simulink library "tqd"  (R2021b)
settings: Solver=VariableStepAuto  StartTime=0.0  StopTime=10.0  RelTol=1e-3
undefined symbols (not defined in the file or in its folder): ATQD_BOSEnBPSPosn_X_kph, ATQD_BOSMap_X_rpm, ATQD_BOSMap_Y_pct, ATQD_CreepBaseTqD_X_kph, ATQD_CreepBaseTqD_Y_Deg, ATQD_CreepBaseTqR_X_kph, ATQD_CreepBaseTqR_Y_Deg, ATQD_CreepBPSDisPosn_X_Deg, ATQD_CreepBPSDisPosnR_X_Deg, ATQD_CreepBPSEnPosn_X_Deg, ATQD_CreepBPSEnPosnR_X_Deg, ATQD_CreepDeltaTq_X_kph, ATQD_CreepIterm_X_kph, ATQD_CreepIterm_Y_kph, ATQD_CreepItermMaxLimit_X_pct, ATQD_CreepPreloadTime_X_kph, ATQD_CreepPreloadTq_X_kph, ATQD_CreepPreloadTq_Y_s, ATQD_CreepProtTq_X_Deg, ATQD_CreepPterm_X_kph, ATQD_ECOTqMapD_X_rpm, ATQD_ECOTqMapD_Y_pct, ATQD_NL1TqMapD_X_rpm, ATQD_NL1TqMapD_Y_pct, ATQD_NRMRrEDUSpRat_X_rpm, ATQD_NRMRrEDUSpRat_Y_Nm, ATQD_PedalMapClimbUpLim_X_rpm, ATQD_PedalMapClimbUpLim_Y_Deg, ATQD_PreLoadTq_X_s, ATQD_SL1TqMapD_X_rpm, ATQD_SL1TqMapD_Y_pct, ATQD_WhlTqCapMotGain_X_pct, ATQD_WhlTqCapMotGain_Y_mV, ENUM_ACCPEDALLOWSW_LOWIDLE, ENUM_ACCPEDALLOWSW_NOIDLE, ENUM_CHRGPLUGSTA_NONE, ENUM_CRASHSTATE_NOCRASH, ENUM_DCDCFAULTSTA_WORKING, ENUM_DRIVEMODE_ECO, ENUM_DRIVEMODE_NRM, ENUM_DRIVEMODE_SPORT, ENUM_DRIVETRAIN_AWD, ENUM_DRIVETRAIN_FWD, ENUM_DRIVETRAIN_RWD, ENUM_EBSBRKSW_PRESSED, ENUM_EBSTORQUERWQ_LIMIT, ENUM_EBSTORQUERWQ_TORQUE, ENUM_EMTRQMODE_ACCL, ENUM_EMTRQMODE_BRAKING, ENUM_EMTRQMODE_COASTING, ENUM_EPBERROR_NORMAL, ENUM_EPBSTA_APPLIED, ENUM_EPBSTA_RELEASED, ENUM_EPBSTA_UNKNOWN, ENUM_EPBSTARAW_NOTSET, ENUM_EPBSTARAW_SET, ENUM_GEARACTUALPOSN_D, ENUM_GEARACTUALPOSN_N, ENUM_GEARACTUALPOSN_P, ENUM_GEARACTUALPOSN_R ... (+201)
libraries: hcu_lib x19, simulink x12
(part 3 of 6)

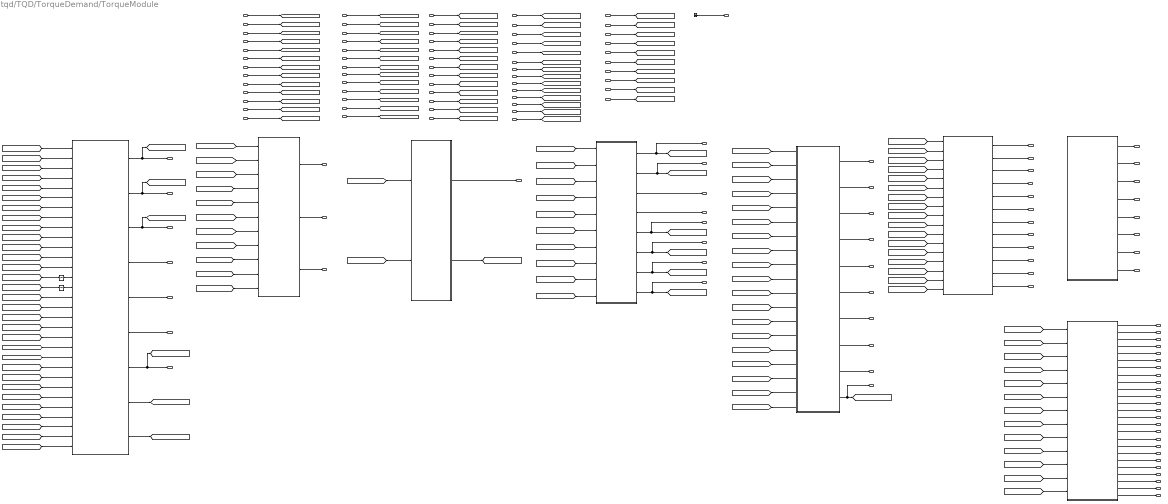
== system tqd/TQD/TorqueDemand/TorqueModule ==
  note: Input Signals
  VTQD_LowIdleAccPedal_flg : Inport
  VPMM_DrivetrainSelect_enum : Inport  Port=2
  VTQD_RollRegenDisableReq_flg : Inport  Port=3
  VTQD_GearActualPosn_enum : Inport  Port=4
  VTQD_CreepON_flg : Inport  Port=5
  VTQD_BrkSwSta_flg : Inport  Port=6
  VTQD_LimpHomeAct_flg : Inport  Port=7
  VTQD_EVDriveMode_enum : Inport  Port=8
  VTQD_RegenMode_enum : Inport  Port=9
  VINP_VehSpeed_kph : Inport  Port=10
  VTQD_TqTargetShaftSpd_rpm : Inport  Port=11
  VTQD_FrShaftSpd_rpm : Inport  Port=12
  VTQD_RrShaftSpd_rpm : Inport  Port=13
  VTQD_ActAPSPosn_pct : Inport  Port=14
  VTQD_ActBPSPosn_pct : Inport  Port=15
  VINP_FrRBCActive_flg : Inport  Port=16
  VINP_RrRBCActive_flg : Inport  Port=17
  VINP_FrntAxlTrqReqBrk_Nm : Inport  Port=18
  VINP_RearAxlTrqReqBrk_Nm : Inport  Port=19
  VINP_HVBPwrAvailDchrg_kw : Inport  Port=20
  VINP_HVBPwrAvailChrg_kw : Inport  Port=21
  VINP_FrRegenAvailTq_Nm : Inport  Port=22
  VINP_RrRegenAvailTq_Nm : Inport  Port=23
  VINP_FrTMSpd_RPM : Inport  Port=24
  VINP_RrTMSpd_RPM : Inport  Port=25
  VINP_FrEDURealTMTq_Nm : Inport  Port=26
  VINP_RrEDURealTMTq_Nm : Inport  Port=27
  VPMM_PwrSta_enum : Inport  Port=28
  VTQD_MCUReady4Ext_flg : Inport  Port=29
  VINP_HVBattErr_flg : Inport  Port=30
  VINP_DCDCFaultSta_enum : Inport  Port=31
  VTQD_TMRotateDirction_enum : Inport  Port=32
  VTQR_ActualFEDUWhlTqReq_Nm : Inport  Port=33
  VTQR_ActualREDUWhlTqReq_Nm : Inport  Port=34
  VTQD_RDCActive_enum : Inport  Port=35
  task_time_s : Inport  Port=36
  VINP_HSAActive_flg : Inport  Port=37
  VTQR_NoABSFEDUWhlTqReq_Nm : Inport  Port=38
  VTQR_NoABSREDUWhlTqReq_Nm : Inport  Port=39
  VINP_EPBErrSta_enum : Inport  Port=40
  VINP_MCUWarnF_enum : Inport  Port=41
  VINP_MCUWarnR_enum : Inport  Port=42
  VVMC_EstSlope_Deg : Inport  Port=43
  VINP_DrDoorSW_flg : Inport  Port=44
  VINP_PsDoorSW_flg : Inport  Port=45
  VINP_RRDoorSW_flg : Inport  Port=46
  VINP_RLDoorSW_flg : Inport  Port=47
  VINP_HoodSW_flg : Inport  Port=48
  VINP_TailgateSW_flg : Inport  Port=49
  VTQD_EPBSta_enum : Inport  Port=50
  VINP_HVBCellVoltMax_mV : Inport  Port=51
  VINP_HVBCellVoltMin_mV : Inport  Port=52
  VINP_HVBSOH_pct : Inport  Port=53
  VINP_HVBattSOC_pct : Inport  Port=54
  VINP_EBSBrakeSW_enum : Inport  Port=55
  VINP_EPBParkingBrakeSta_enum : Inport  Port=56
  VTQR_RampREDUWhlTqReq_Nm : Inport  Port=57
  VTQD_EM1ReqTorqLimBrk_Nm : Inport  Port=58
  VTQD_EM1ReqTorqLimDriv_Nm : Inport  Port=59
  VTQD_EM1TorqueCtrlBrk_flg : Inport  Port=60
  VTQD_EM1LimitCtrlBrk_flg : Inport  Port=61
  VTQD_EM1TorqueCtrlDriv_flg : Inport  Port=62
  VTQD_EM1LimitCtrlDriv_flg : Inport  Port=63
  AvaliableTqLimit : Subsystem
  DriverWhlTqDem : Subsystem
  ExtTqFuncHandShaking : Subsystem
  Ground : Ground
  Signal for ESC : Subsystem
  Signals for MCU : Subsystem
  TQD Output Signal Convert : Subsystem
  TqCoordination : Subsystem
  TqDistribution : Subsystem
  Unit Delay : UnitDelay  SampleTime=-1  HasFrameUpgradeWarning=on
  Unit Delay1 : UnitDelay  SampleTime=-1  HasFrameUpgradeWarning=on
  VTQD_DriverWhlTqDem_Nm : Outport
  VTQD_TqSourceFr_enum : Outport  Port=2
  VTQD_TqSourceRr_enum : Outport  Port=3
  VTQD_RollRegenEnable_flg : Outport  Port=4
  VTQD_AfterAvailableTqDemFr_Nm : Outport  Port=5
  VTQD_AfterAvailableTqDemRr_Nm : Outport  Port=6
  VTQD_FrEDUAvailBrkRgnTq_Nm : Outport  Port=7
  VTQD_RrEDUAvailBrkRgnTq_Nm : Outport  Port=8
  VTQD_FrRgnDecrSta_flg : Outport  Port=9
  VTQD_RrRgnDecrSta_flg : Outport  Port=10
  VTQD_FrEDUActTq_Nm : Outport  Port=11
  VTQD_RrEDUActTq_Nm : Outport  Port=12
  VTQD_FrEDURolRgnTq_Nm : Outport  Port=13
  VTQD_RrEDURolRgnTq_Nm : Outport  Port=14
  VTQD_FrEDUSpd_rpm : Outport  Port=15
  VTQD_RrEDUSpd_rpm : Outport  Port=16
  VTQD_FrEDUSpdValid_flg : Outport  Port=17
  VTQD_FrEDUAvailBrkRgnTqV_flg : Outport  Port=18
  VTQD_RrEDUSpdValid_flg : Outport  Port=19
  VTQD_RrEDUAvailBrkRgnTqV_flg : Outport  Port=20
  VTQD_RgnAbnorSta_flg : Outport  Port=21
  VTQD_PTCSPermSta_flg : Outport  Port=22
  VTQD_FrRgnPermSta_flg : Outport  Port=23
  VTQD_RrRgnPermSta_flg : Outport  Port=24
  VTQD_DriverWhlTqDemFr_Nm : Outport  Port=25
  VTQD_DriverWhlTqDemRr_Nm : Outport  Port=26
  VTQD_ExternalTqAllow_flg : Outport  Port=27
  VTQD_FrIdcMin_A : Outport  Port=28
  VTQD_FrIdcMax_A : Outport  Port=29
  VTQD_FrUdcMin_V : Outport  Port=30
  VTQD_FrUdcMax_V : Outport  Port=31
  VTQD_RrIdcMin_A : Outport  Port=32
  VTQD_RrIdcMax_A : Outport  Port=33
  VTQD_RrUdcMin_V : Outport  Port=34
  VTQD_RrUdcMax_V : Outport  Port=35
  VTQD_CoordWhlTqDemFr_Nm : Outport  Port=36
  VTQD_CoordWhlTqDemRr_Nm : Outport  Port=37
  VTQD_CreepEnable_flg : Outport  Port=38
  VTQD_ReBrakeLPReq_flg : Outport  Port=39
  VTQD_BOSEnable_flg : Outport  Port=40
  VTQD_ExtShftAllow_flg : Outport  Port=41
  VTQD_PreLoadHold_flg : Outport  Port=42
  VTQD_PreLoadPreEn_flg : Outport  Port=43
  VTQD_CreepPrLoadEnable_flg : Outport  Port=44
  VTQD_ExtDoorAllow_flg : Outport  Port=45
  VTQD_WhlTqCapGenFr_Nm : Outport  Port=46
  VTQD_WhlTqCapGenRr_Nm : Outport  Port=47
  VTQD_ActEMpTrq_pct : Outport  Port=48
  VTQD_ActMaxAvaEMRecpTrq_pct : Outport  Port=49
  VTQD_ActDriveDirect_enum : Outport  Port=50
  VTQD_DLEngaged_enum : Outport  Port=51
  VTQD_EMTrqModeDrvBrk_enum : Outport  Port=52
  VTQD_ActEMpTrqHrls_pct : Outport  Port=53
  VTQD_ActEMOutSftSpd_rpm : Outport  Port=54
  VTQD_DrvDemEMRtapTrq_pct : Outport  Port=55
  VTQD_SACtrlDev_enum : Outport  Port=56
  VTQD_RetSelNonEng_pct : Outport  Port=57
  VTQD_ShiftPgs_enum : Outport  Port=58
  VTQD_AccPedal1LowSW_enum : Outport  Port=59
  VTQD_AccPedalPos1_pct : Outport  Port=60
  VTQD_ParkBrakeSW_enum : Outport  Port=61
  VTQD_VCUVehSpd_kph : Outport  Port=62
  VTQD_BrakeSW_enum : Outport  Port=63
  VTQD_NFricPercTorq_pct : Outport  Port=64
  VTQD_EMParasLoss_pct : Outport  Port=65
  VTQD_EEC2MSGCnt_raw : Outport  Port=66
  VTQD_EEC2MSGCS_raw : Outport  Port=67
  VTQD_FDCCHAEBSRd4BRSta_enum : Outport  Port=68
  VTQD_FDCCHAEBSHBSwSta_enum : Outport  Port=69
  VTQD_FDCCHAEBSHHSwSta_enum : Outport  Port=70
  VTQD_FDCVCUTUpAStaSta_enum : Outport  Port=71
  VTQD_FDCVCUDACStatusSta_enum : Outport  Port=72
  VTQD_CoordTqDem_Nm : Outport  Port=73
  VTQD_FrEDUSpRat_rat : Outport  Port=74
  VTQD_RrEDUSpRat_rat : Outport  Port=75
  wires:
  VTQD_ActAPSPosn_pct/1 -> [VTQD_ActAPSPosn_pct]
  VTQD_GearActualPosn_enum/1 -> [VTQD_GearActualPosn_enum]
  VINP_VehSpeed_kph/1 -> [VINP_VehSpeed_kph]
  VTQD_BrkSwSta_flg/1 -> [VTQD_BrkSwSta_flg]
  VTQD_RegenMode_enum/1 -> [VTQD_RegenMode_enum]
  VINP_FrntAxlTrqReqBrk_Nm/1 -> [VINP_FrntAxlTrqReqBrk_Nm]
  VINP_RearAxlTrqReqBrk_Nm/1 -> [VINP_RearAxlTrqReqBrk_Nm]
  VTQD_RollRegenDisableReq_flg/1 -> [VTQD_RollRegenDisableReq_flg]
  VINP_FrRBCActive_flg/1 -> [VINP_FrRBCActive_flg]
  VTQD_ActBPSPosn_pct/1 -> [VTQD_ActBPSPosn_pct]
  VTQD_EVDriveMode_enum/1 -> [VTQD_EVDriveMode_enum]
  VTQD_LimpHomeAct_flg/1 -> [VTQD_LimpHomeAct_flg]
  VTQD_CreepON_flg/1 -> [VTQD_CreepON_flg]
  VTQD_TqTargetShaftSpd_rpm/1 -> [VTQD_TqTargetShaftSpd_rpm]
  VPMM_DrivetrainSelect_enum/1 -> [VPMM_DrivetrainSelect_enum]
  [VTQD_TqTargetShaftSpd_rpm] -> DriverWhlTqDem/10(VTQD_TqTargetShaftSpd_rpm)
  [VTQD_LimpHomeAct_flg] -> DriverWhlTqDem/6(VTQD_LimpHomeAct_flg)
  [VTQD_EVDriveMode_enum] -> DriverWhlTqDem/7(VTQD_EVDriveMode_enum)
  [VTQD_RegenMode_enum] -> DriverWhlTqDem/8(VTQD_RegenMode_enum)
  [VTQD_CreepON_flg] -> DriverWhlTqDem/4("VTQD_CreepON_flg ")
  [VTQD_GearActualPosn_enum] -> DriverWhlTqDem/3(VTQD_GearActualPosn_enum)
  [VTQD_LowIdleAccPedal_flg] -> DriverWhlTqDem/1(VDHP_LowIdleAccPedal_flg)
  [VTQD_ActAPSPosn_pct] -> DriverWhlTqDem/11(VTQD_ActAPSPosn_pct)
  TqDistribution/2(VTQD_RrEDUSpRat_rat) -> VTQD_RrEDUSpRat_rat/1, [VTQD_RrEDUSpRat_rat]
  TqDistribution/1(VTQD_FrEDUSpRat_rat) -> VTQD_FrEDUSpRat_rat/1, [VTQD_FrEDUSpRat_rat]
  VINP_HVBPwrAvailChrg_kw/1 -> [VINP_HVBPwrAvailChrg_kw]
  VINP_HVBPwrAvailDchrg_kw/1 -> [VINP_HVBPwrAvailDchrg_kw]
  DriverWhlTqDem/1(VTQD_DriverWhlTqDem_Nm) -> [VTQD_DriverWhlTqDem_Nm], VTQD_DriverWhlTqDem_Nm/1
  [VPMM_DrivetrainSelect_enum] -> TqDistribution/1(VPMM_DrivetrainSelect_enum)
  [VTQD_BrkSwSta_flg] -> DriverWhlTqDem/5(VTQD_BrkSwSta_flg)
  [VTQD_ActBPSPosn_pct] -> DriverWhlTqDem/12(VTQD_ActBPSPosn_pct)
  [VINP_VehSpeed_kph] -> DriverWhlTqDem/9(VINP_VehSpeed_kph)
  [VTQD_RollRegenDisableReq_flg] -> DriverWhlTqDem/2(VTQD_RollRegenDisableReq_flg)
  VTQD_FrShaftSpd_rpm/1 -> [VTQD_FrShaftSpd_rpm]
  VTQD_RrShaftSpd_rpm/1 -> [VTQD_RrShaftSpd_rpm]
  VTQD_LowIdleAccPedal_flg/1 -> [VTQD_LowIdleAccPedal_flg]
  DriverWhlTqDem/2(VTQD_RollRegenEnable_flg) -> [VTQD_RollRegenEnable_flg], VTQD_RollRegenEnable_flg/1
  VINP_RrRBCActive_flg/1 -> [VINP_RrRBCActive_flg]
  VINP_RrTMSpd_RPM/1 -> [VINP_RrTMSpd_rpm]
  VINP_FrTMSpd_RPM/1 -> [VINP_FrTMSpd_rpm]
  VINP_RrRegenAvailTq_Nm/1 -> [VINP_RrRegenAvailTq_Nm]
  VINP_FrRegenAvailTq_Nm/1 -> [VINP_FrRegenAvailTq_Nm]
  VINP_RrEDURealTMTq_Nm/1 -> [VINP_RrEDURealTMTq_Nm]
  VINP_FrEDURealTMTq_Nm/1 -> [VINP_FrEDURealTMTq_Nm]
  AvaliableTqLimit/8(VTQD_RrRgnPermSta_flg) -> VTQD_RrRgnPermSta_flg/1  "VTQD_RrRgnPermSta_flg"
  AvaliableTqLimit/6(VTQD_RrRgnDecrSta_flg) -> VTQD_RrRgnDecrSta_flg/1  "VTQD_RrRgnDecrSta_flg"
  Signal for ESC/4(VTQD_RrEDURolRgnTq_Nm) -> VTQD_RrEDURolRgnTq_Nm/1
  AvaliableTqLimit/7(VTQD_FrRgnPermSta_flg) -> VTQD_FrRgnPermSta_flg/1  "VTQD_FrRgnPermSta_flg"
  [VTQD_RrShaftSpd_rpm] -> AvaliableTqLimit/2(VTQD_RrShaftSpd_rpm)
  Signal for ESC/2(VTQD_RrEDUActTq_Nm) -> VTQD_RrEDUActTq_Nm/1
  Signal for ESC/12(VTQD_PTCSPermSta_flg) -> VTQD_PTCSPermSta_flg/1
  Signal for ESC/6(VTQD_RrEDUSpd_rpm) -> VTQD_RrEDUSpd_rpm/1
  Signal for ESC/1(VTQD_FrEDUActTq_Nm) -> VTQD_FrEDUActTq_Nm/1
  [VINP_RrRegenAvailTq_Nm] -> AvaliableTqLimit/12(VINP_RrRegenAvailTq_Nm)
  [VINP_HVBPwrAvailChrg_kw] -> AvaliableTqLimit/4(VINP_HVBPwrAvailChrg_kw)
  [VTQD_FrShaftSpd_rpm] -> AvaliableTqLimit/1(VTQD_FrShaftSpd_rpm)
  AvaliableTqLimit/1(VTQD_AfterAvailableTqDemFr_Nm) -> VTQD_AfterAvailableTqDemFr_Nm/1
  [VINP_HVBPwrAvailDchrg_kw] -> AvaliableTqLimit/3(VINP_HVBPwrAvailDchrg_kw)
  Signal for ESC/11(VTQD_RgnAbnorSta_flg) -> VTQD_RgnAbnorSta_flg/1
  Signal for ESC/9(VTQD_RrEDUSpdValid_flg) -> VTQD_RrEDUSpdValid_flg/1  "VTQD_RrEDUSpdValid_flg"
  Signal for ESC/3(VTQD_FrEDURolRgnTq_Nm) -> VTQD_FrEDURolRgnTq_Nm/1
  [VINP_FrRegenAvailTq_Nm] -> AvaliableTqLimit/11(VINP_FrRegenAvailTq_Nm)
  AvaliableTqLimit/5(VTQD_FrRgnDecrSta_flg) -> VTQD_FrRgnDecrSta_flg/1  "VTQD_FrRgnDecrSta_flg"
  AvaliableTqLimit/2(VTQD_AfterAvailableTqDemRr_Nm) -> VTQD_AfterAvailableTqDemRr_Nm/1
  AvaliableTqLimit/3(VTQD_FrEDUAvailBrkRgnTq_Nm) -> VTQD_FrEDUAvailBrkRgnTq_Nm/1
  [VTQR_ActualREDUWhlTqReq_Nm] -> AvaliableTqLimit/6(VTQR_ActualREDUWhlTqReq_Nm)
  Signal for ESC/10(VTQD_RrEDUAvailBrkRgnTqV_flg) -> VTQD_RrEDUAvailBrkRgnTqV_flg/1  "VTQD_RrEDUAvailBrkRgnTqV_flg"
  [VTQD_DriverWhlTqDemFr_Nm] -> AvaliableTqLimit/9(VTQD_DriverWhlTqDemFr_Nm)
  [VTQR_ActualFEDUWhlTqReq_Nm] -> AvaliableTqLimit/5(VTQR_ActualFEDUWhlTqReq_Nm)
  [VTQD_DriverWhlTqDemRr_Nm] -> AvaliableTqLimit/10(VTQD_DriverWhlTqDemRr_Nm)
  [VTQD_FrEDUSpRat_rat] -> AvaliableTqLimit/7(VTQD_FrEDUSpRat_rat)
  [VTQD_RrEDUSpRat_rat] -> AvaliableTqLimit/8(VTQD_RrEDUSpRat_rat)
  Signal for ESC/5(VTQD_FrEDUSpd_rpm) -> VTQD_FrEDUSpd_rpm/1
  AvaliableTqLimit/4(VTQD_RrEDUAvailBrkRgnTq_Nm) -> VTQD_RrEDUAvailBrkRgnTq_Nm/1
  Signal for ESC/7(VTQD_FrEDUSpdValid_flg) -> VTQD_FrEDUSpdValid_flg/1  "VTQD_FrEDUSpdValid_flg"
  [VINP_DCDCFaultSta_enum] -> ExtTqFuncHandShaking/4(VINP_DCDCFaultSta_enum)
  [VINP_HVBattErr_flg] -> ExtTqFuncHandShaking/3(VINP_HVBattErr_flg)
  [VTQD_MCUReady4Ext_flg] -> ExtTqFuncHandShaking/2(VTQD_MCUReady4Ext_flg)
  [VPMM_PwrSta_enum] -> ExtTqFuncHandShaking/1(VPMM_PwrSta_enum)
  VINP_HVBattErr_flg/1 -> [VINP_HVBattErr_flg]
  VTQD_MCUReady4Ext_flg/1 -> [VTQD_MCUReady4Ext_flg]
  VPMM_PwrSta_enum/1 -> [VPMM_PwrSta_enum]
  VINP_DCDCFaultSta_enum/1 -> [VINP_DCDCFaultSta_enum]
  ExtTqFuncHandShaking/1(VTQD_ExternalTqAllow_flg) -> VTQD_ExternalTqAllow_flg/1
  VTQD_TMRotateDirction_enum/1 -> [VTQD_TMRotateDirction_enum]
  [VTQD_TMRotateDirction_enum] -> DriverWhlTqDem/13(VTQD_TMRotateDirction_enum)
  Signals for MCU/8(VTQD_RrUdcMax_V) -> VTQD_RrUdcMax_V/1
  Signals for MCU/5(VTQD_RrIdcMin_A) -> VTQD_RrIdcMin_A/1
  Signals for MCU/3(VTQD_FrUdcMin_V) -> VTQD_FrUdcMin_V/1
  Signals for MCU/2(VTQD_FrIdcMax_A) -> VTQD_FrIdcMax_A/1
  Signals for MCU/7(VTQD_RrUdcMin_V) -> VTQD_RrUdcMin_V/1
  Signals for MCU/6(VTQD_RrIdcMax_A) -> VTQD_RrIdcMax_A/1
  Signals for MCU/4(VTQD_FrUdcMax_V) -> VTQD_FrUdcMax_V/1
  Signals for MCU/1(VTQD_FrIdcMin_A) -> VTQD_FrIdcMin_A/1
  [VTQD_TqSourceFr_enum] -> Unit Delay/1
  [VTQD_TqSourceRr_enum] -> Unit Delay1/1
  Unit Delay/1 -> DriverWhlTqDem/14(VTQD_TqSourceFr_enum)
  Unit Delay1/1 -> DriverWhlTqDem/15(VTQD_TqSourceRr_enum)
  DriverWhlTqDem/3(VTQD_CreepEnable_flg) -> [VTQD_CreepEnable_flg], VTQD_CreepEnable_flg/1
  [VTQD_DriverWhlTqDem_Nm] -> AvaliableTqLimit/13(VTQD_DriverWhlTqDem_Nm)
  Ground/1 -> VTQD_ReBrakeLPReq_flg/1  "VTQD_ReBrakeLPReq_flg"
  VTQR_ActualFEDUWhlTqReq_Nm/1 -> [VTQR_ActualFEDUWhlTqReq_Nm]
  VTQR_ActualREDUWhlTqReq_Nm/1 -> [VTQR_ActualREDUWhlTqReq_Nm]
  VTQD_RDCActive_enum/1 -> [VTQD_RDCActive_enum]
  [VTQD_RDCActive_enum] -> DriverWhlTqDem/16(VTQD_RDCActive_enum)
  [VTQD_CreepEnable_flg] -> AvaliableTqLimit/14(VTQD_CreepEnable_flg)
  [VINP_FrEDURealTMTq_Nm] -> Signal for ESC/1(VINP_FrEDURealTMTq_Nm)
  [VINP_RrEDURealTMTq_Nm] -> Signal for ESC/2(VINP_RrEDURealTMTq_Nm)
  [VTQD_RollRegenEnable_flg] -> Signal for ESC/3(VTQD_RollRegenEnable_flg)
  [VINP_MCUWarnR_enum] -> Signal for ESC/9(VINP_MCUWarnR_enum)
  [VINP_MCUWarnF_enum] -> Signal for ESC/8(VINP_MCUWarnF_enum)
  [VTQD_GearActualPosn_enum] -> TqCoordination/1(VTQD_GearActualPosn_enum)
  [VTQD_DriverWhlTqDem_Nm] -> TqCoordination/2(VTQD_DriverWhlTqDem_Nm)
  task_time_s/1 -> [task_time_s]
  [task_time_s] -> DriverWhlTqDem/17(task_time_s)
  Signal for ESC/8(VTQD_FrEDUAvailBrkRgnTqV_flg) -> VTQD_FrEDUAvailBrkRgnTqV_flg/1  "VTQD_FrEDUAvailBrkRgnTqV_flg"
  DriverWhlTqDem/4(VTQD_BOSEnable_flg) -> VTQD_BOSEnable_flg/1
  VINP_HSAActive_flg/1 -> [VINP_HSAActive_flg]
  VTQR_NoABSFEDUWhlTqReq_Nm/1 -> [VTQR_NoABSFEDUWhlTqReq_Nm]
  VTQR_NoABSREDUWhlTqReq_Nm/1 -> [VTQR_NoABSREDUWhlTqReq_Nm]
  VINP_MCUWarnF_enum/1 -> [VINP_MCUWarnF_enum]
  VINP_MCUWarnR_enum/1 -> [VINP_MCUWarnR_enum]
  VINP_EPBErrSta_enum/1 -> [VINP_EPBErrSta_enum]
  [VINP_HSAActive_flg] -> DriverWhlTqDem/18(VINP_HSAActive_flg)
  [VINP_RrRBCActive_flg] -> DriverWhlTqDem/19(VINP_RrRBCActive_flg)
  [VINP_FrRBCActive_flg] -> DriverWhlTqDem/20(VINP_FrRBCActive_flg)
  [VINP_EPBErrSta_enum] -> ExtTqFuncHandShaking/5(VINP_EPBErrSta_enum)
  ExtTqFuncHandShaking/2(VTQD_ExtShftAllow_flg) -> VTQD_ExtShftAllow_flg/1
  [VINP_FrntAxlTrqReqBrk_Nm] -> Signal for ESC/4(VINP_FrntAxlTrqReqBrk_Nm)
  [VINP_RearAxlTrqReqBrk_Nm] -> Signal for ESC/5(VINP_RearAxlTrqReqBrk_Nm)
  [VINP_FrRBCActive_flg] -> Signal for ESC/10(VINP_FrRBCActive_flg)
  [VINP_RrRBCActive_flg] -> Signal for ESC/11(VINP_RrRBCActive_flg)
  [VTQR_ActualFEDUWhlTqReq_Nm] -> Signal for ESC/12(VTQR_ActualFEDUWhlTqReq_Nm)
  [VTQR_ActualREDUWhlTqReq_Nm] -> Signal for ESC/13(VTQR_ActualREDUWhlTqReq_Nm)
  [VTQR_NoABSFEDUWhlTqReq_Nm] -> Signal for ESC/14(VTQR_NoABSFEDUWhlTqReq_Nm)
  [VTQR_NoABSREDUWhlTqReq_Nm] -> Signal for ESC/15(VTQR_NoABSREDUWhlTqReq_Nm)
  [VTQD_DriverWhlTqDem_Nm] -> Signal for ESC/16(VTQD_DriverWhlTqDem_Nm)
  [VINP_FrTMSpd_rpm] -> Signal for ESC/6(VINP_FrTMSpd_rpm)
  [VINP_RrTMSpd_rpm] -> Signal for ESC/7(VINP_RrTMSpd_rpm)
  [VINP_FrEDURealTMTq_Nm] -> DriverWhlTqDem/21(VINP_FrEDURealTMTq_Nm)
  [VINP_RrEDURealTMTq_Nm] -> DriverWhlTqDem/22(VINP_RrEDURealTMTq_Nm)
  DriverWhlTqDem/6(VTQD_PreLoadPreEn_flg) -> VTQD_PreLoadPreEn_flg/1
  DriverWhlTqDem/7(VTQD_CreepPrLoadEnable_flg) -> [VTQD_CreepPrLoadEnable_flg], VTQD_CreepPrLoadEnable_flg/1
  DriverWhlTqDem/5(VTQD_PreLoadHold_flg) -> VTQD_PreLoadHold_flg/1
  [VTQD_RrShaftSpd_rpm] -> TqDistribution/2(VTQD_RrShaftSpd_rpm)
  [VTQD_DriverWhlTqDem_Nm] -> TqDistribution/3(VTQD_DriverWhlTqDem_Nm)
  [VTQD_EVDriveMode_enum] -> TqDistribution/4(VTQD_EVDriveMode_enum)
  [VTQD_LimpHomeAct_flg] -> TqDistribution/5(VTQD_LimpHomeAct_flg)
  [VTQD_CreepPrLoadEnable_flg] -> TqDistribution/6(VTQD_CreepPrLoadEnable_flg)
  VVMC_EstSlope_Deg/1 -> [VVMC_EstSlope_Deg]
  [VVMC_EstSlope_Deg] -> DriverWhlTqDem/23(VVMC_EstSlope_Deg)
  [VPMM_PwrSta_enum] -> DriverWhlTqDem/24(VPMM_PwrSta_enum)
  [VINP_EPBSta_enum] -> DriverWhlTqDem/25(VINP_EPBSta_enum)
  DriverWhlTqDem/8(VTQD_VehActSpd_kph) -> [VTQD_VehActSpd_kph]
  [VINP_DrDoorSW_flg] -> ExtTqFuncHandShaking/6(VINP_DrDoorSW_flg)
  [VINP_PsDoorSW_flg] -> ExtTqFuncHandShaking/7(VINP_PsDoorSW_flg)
  [VINP_RRDoorSW_flg] -> ExtTqFuncHandShaking/8(VINP_RRDoorSW_flg)
  [VINP_RLDoorSW_flg] -> ExtTqFuncHandShaking/9(VINP_RLDoorSW_flg)
  [VINP_HoodSW_flg] -> ExtTqFuncHandShaking/10(VINP_HoodSW_flg)
  [VINP_TailgateSW_flg] -> ExtTqFuncHandShaking/11(VINP_TailgateSW_flg)
  ExtTqFuncHandShaking/3(VTQD_ExtDoorAllow_flg) -> VTQD_ExtDoorAllow_flg/1
  TqCoordination/1(VTQD_CoordTqDem_Nm) -> VTQD_CoordTqDem_Nm/1
  TqCoordination/2(VTQD_TqSource_enum) -> [VTQD_TqSource_enum]
  [VTQD_TqSource_enum] -> TqDistribution/8(VTQD_TqSource_enum)
  TqDistribution/3(VTQD_CoordWhlTqDemFr_Nm) -> VTQD_CoordWhlTqDemFr_Nm/1
  TqDistribution/4(VTQD_CoordWhlTqDemRr_Nm) -> VTQD_CoordWhlTqDemRr_Nm/1
  TqDistribution/5(VTQD_TqSourceFr_enum) -> VTQD_TqSourceFr_enum/1, [VTQD_TqSourceFr_enum]
  TqDistribution/6(VTQD_TqSourceRr_enum) -> VTQD_TqSourceRr_enum/1, [VTQD_TqSourceRr_enum]
  TqDistribution/7(VTQD_DriverWhlTqDemFr_Nm) -> VTQD_DriverWhlTqDemFr_Nm/1, [VTQD_DriverWhlTqDemFr_Nm]
  TqDistribution/8(VTQD_DriverWhlTqDemRr_Nm) -> VTQD_DriverWhlTqDemRr_Nm/1, [VTQD_DriverWhlTqDemRr_Nm]
  VINP_RLDoorSW_flg/1 -> [VINP_RLDoorSW_flg]
  VINP_HoodSW_flg/1 -> [VINP_HoodSW_flg]
  VINP_TailgateSW_flg/1 -> [VINP_TailgateSW_flg]
  VINP_DrDoorSW_flg/1 -> [VINP_DrDoorSW_flg]
  VINP_PsDoorSW_flg/1 -> [VINP_PsDoorSW_flg]
  VINP_RRDoorSW_flg/1 -> [VINP_RRDoorSW_flg]
  VTQD_EPBSta_enum/1 -> [VINP_EPBSta_enum]
  [VTQD_VehActSpd_kph] -> AvaliableTqLimit/15(VTQD_VehActSpd_kph)
  VINP_HVBSOH_pct/1 -> [VINP_HVBSOH_pct]
  VINP_HVBCellVoltMax_mV/1 -> [VINP_HVBCellVoltMax_mV]
  VINP_HVBCellVoltMin_mV/1 -> [VINP_HVBCellVoltMin_mV]
  [VINP_HVBSOH_pct] -> AvaliableTqLimit/18(VINP_HVBSOH_pct)
  [VINP_HVBCellVoltMin_mV] -> AvaliableTqLimit/17(VINP_HVBCellVoltMin_mV)
  [VINP_HVBCellVoltMax_mV] -> AvaliableTqLimit/16(VINP_HVBCellVoltMax_mV)
  AvaliableTqLimit/9(VTQD_WhlTqCapGenFr_Nm) -> VTQD_WhlTqCapGenFr_Nm/1
  AvaliableTqLimit/10(VTQD_WhlTqCapGenRr_Nm) -> VTQD_WhlTqCapGenRr_Nm/1, [VTQD_WhlTqCapGenRr_Nm]
  VINP_HVBattSOC_pct/1 -> [VINP_HVBattSOC_pct]
  [VINP_HVBattSOC_pct] -> Signal for ESC/17(VINP_HVBattSOC_pct)
  [VTQD_RollRegenEnable_flg] -> TQD Output Signal Convert/1(VTQD_RollRegenEnable_flg)
  [VTQD_GearActualPosn_enum] -> TQD Output Signal Convert/2(VTQD_GearActualPosn_enum)
  [VINP_RrEDURealTMTq_Nm] -> TQD Output Signal Convert/3(VINP_RrEDURealTMTq_Nm)
  [VTQD_WhlTqCapGenRr_Nm] -> TQD Output Signal Convert/4(VTQD_WhlTqCapGenRr_Nm)
  [VINP_RrRegenAvailTq_Nm] -> TQD Output Signal Convert/5(VINP_RrRegenAvailTq_Nm)
  [VPMM_PwrSta_enum] -> TQD Output Signal Convert/6(VPMM_PwrSta_enum)
  TQD Output Signal Convert/3(VTQD_ActEMpTrq_pct) -> VTQD_ActEMpTrq_pct/1
  TQD Output Signal Convert/8(VTQD_ActMaxAvaEMRecpTrq_pct) -> VTQD_ActMaxAvaEMRecpTrq_pct/1
  TQD Output Signal Convert/9(VTQD_ActDriveDirect_enum) -> VTQD_ActDriveDirect_enum/1
  TQD Output Signal Convert/10(VTQD_DLEngaged_enum) -> VTQD_DLEngaged_enum/1
  [VINP_RrTMSpd_rpm] -> TQD Output Signal Convert/7(VINP_RrTMSpd_rpm)
  [VTQD_ActAPSPosn_pct] -> TQD Output Signal Convert/8(VTQD_ActAPSPosn_pct)
  [VTQD_LowIdleAccPedal_flg] -> TQD Output Signal Convert/9(VTQD_LowIdleAccPedal_flg)
  [VINP_VehSpeed_kph] -> TQD Output Signal Convert/10(VINP_VehSpeed_kph)
  [VINP_EBSBrakeSW_enum] -> TQD Output Signal Convert/11(VINP_EBSBrakeSW_enum)
  [VINP_EPBParkingBrakeSta_enum] -> TQD Output Signal Convert/12(VINP_EPBParkingBrakeSta_enum)
  [VTQD_PedalMapWhlTq_Nm] -> TQD Output Signal Convert/13(VTQD_PedalMapWhlTq_Nm)
  TQD Output Signal Convert/1(VTQD_EMTrqModeDrvBrk_enum) -> VTQD_EMTrqModeDrvBrk_enum/1
  TQD Output Signal Convert/2(VTQD_ActEMpTrqHrls_pct) -> VTQD_ActEMpTrqHrls_pct/1
  TQD Output Signal Convert/4(VTQD_ActEMOutSftSpd_rpm) -> VTQD_ActEMOutSftSpd_rpm/1
  TQD Output Signal Convert/5(VTQD_DrvDemEMRtapTrq_pct) -> VTQD_DrvDemEMRtapTrq_pct/1
  TQD Output Signal Convert/6(VTQD_SACtrlDev_enum) -> VTQD_SACtrlDev_enum/1
  TQD Output Signal Convert/7(VTQD_RetSelNonEng_pct) -> VTQD_RetSelNonEng_pct/1
  TQD Output Signal Convert/18(VTQD_EMParasLoss_pct) -> VTQD_EMParasLoss_pct/1
  TQD Output Signal Convert/11(VTQD_ShiftPgs_enum) -> VTQD_ShiftPgs_enum/1
  TQD Output Signal Convert/12(VTQD_AccPedal1LowSW_enum) -> VTQD_AccPedal1LowSW_enum/1
  TQD Output Signal Convert/13(VTQD_AccPedalPos1_pct) -> VTQD_AccPedalPos1_pct/1
  TQD Output Signal Convert/14(VTQD_ParkBrakeSW_enum) -> VTQD_ParkBrakeSW_enum/1
  TQD Output Signal Convert/15(VTQD_VCUVehSpd_kph) -> VTQD_VCUVehSpd_kph/1
  TQD Output Signal Convert/16(VTQD_BrakeSW_enum) -> VTQD_BrakeSW_enum/1
  TQD Output Signal Convert/17(VTQD_NFricPercTorq_pct) -> VTQD_NFricPercTorq_pct/1
  VINP_EBSBrakeSW_enum/1 -> [VINP_EBSBrakeSW_enum]
  VINP_EPBParkingBrakeSta_enum/1 -> [VINP_EPBParkingBrakeSta_enum]
  TQD Output Signal Convert/19(VTQD_EEC2MSGCnt_raw) -> VTQD_EEC2MSGCnt_raw/1
  TQD Output Signal Convert/20(VTQD_EEC2MSGCS_raw) -> VTQD_EEC2MSGCS_raw/1
  TQD Output Signal Convert/21(VTQD_FDCCHAEBSRd4BRSta_enum) -> VTQD_FDCCHAEBSRd4BRSta_enum/1
  TQD Output Signal Convert/22(VTQD_FDCCHAEBSHBSwSta_enum) -> VTQD_FDCCHAEBSHBSwSta_enum/1
  TQD Output Signal Convert/23(VTQD_FDCCHAEBSHHSwSta_enum) -> VTQD_FDCCHAEBSHHSwSta_enum/1
  TQD Output Signal Convert/24(VTQD_FDCVCUTUpAStaSta_enum) -> VTQD_FDCVCUTUpAStaSta_enum/1
  TQD Output Signal Convert/25(VTQD_FDCVCUDACStatusSta_enum) -> VTQD_FDCVCUDACStatusSta_enum/1
  VTQR_RampREDUWhlTqReq_Nm/1 -> [VTQR_RampREDUWhlTqReq_Nm]
  [VTQR_RampREDUWhlTqReq_Nm] -> TqDistribution/7(VTQR_RampREDUWhlTqReq_Nm)
  [VTQD_GearActualPosn_enum] -> AvaliableTqLimit/19(VTQD_GearActualPosn_enum)
  VTQD_EM1LimitCtrlBrk_flg/1 -> [VTQD_EM1LimitCtrlBrk_flg]
  VTQD_EM1TorqueCtrlBrk_flg/1 -> [VTQD_EM1TorqueCtrlBrk_flg]
  VTQD_EM1ReqTorqLimDriv_Nm/1 -> [VTQD_EM1ReqTorqLimDriv_Nm]
  VTQD_EM1ReqTorqLimBrk_Nm/1 -> [VTQD_EM1ReqTorqLimBrk_Nm]
  VTQD_EM1TorqueCtrlDriv_flg/1 -> [VTQD_EM1TorqueCtrlDriv_flg]
  VTQD_EM1LimitCtrlDriv_flg/1 -> [VTQD_EM1LimitCtrlDriv_flg]
  [VTQD_EM1ReqTorqLimBrk_Nm] -> DriverWhlTqDem/26(VTQD_EM1ReqTorqLimBrk_Nm)
  [VTQD_EM1ReqTorqLimDriv_Nm] -> DriverWhlTqDem/27(VTQD_EM1ReqTorqLimDriv_Nm)
  [VTQD_EM1TorqueCtrlBrk_flg] -> DriverWhlTqDem/28(VTQD_EM1TorqueCtrlBrk_flg)
  [VTQD_EM1LimitCtrlBrk_flg] -> DriverWhlTqDem/29(VTQD_EM1LimitCtrlBrk_flg)
  [VTQD_EM1TorqueCtrlDriv_flg] -> DriverWhlTqDem/30(VTQD_EM1TorqueCtrlDriv_flg)
  [VTQD_EM1LimitCtrlDriv_flg] -> DriverWhlTqDem/31(VTQD_EM1LimitCtrlDriv_flg)
  [VTQD_EM1TorqueCtrlDriv_flg] -> TqDistribution/10(VTQD_EM1TorqueCtrlDriv_flg)
  [VTQD_EM1TorqueCtrlBrk_flg] -> TqDistribution/9(VTQD_EM1TorqueCtrlBrk_flg)
  DriverWhlTqDem/9(VTQD_PedalMapWhlTq_Nm) -> [VTQD_PedalMapWhlTq_Nm]

== system tqd/TQD/TorqueDemand/ShiftModule/GearShiftPosn ==
  VINP_ShifterHandleCmd_enum : Inport
  VPMM_PowerSta_enum : Inport  Port=2
  VINP_VehSpeed_kph : Inport  Port=3
  VINP_ChrgPlugSta_enum : Inport  Port=4
  AND5 : Logic  Inputs=4  AllPortsSameDT=off  OutDataTypeStr=boolean
  Constant : Constant  Value=ENUM_GEARSHIFTCMD_R
  Constant1 : Constant  Value=ENUM_POWERSTA_READY
  Constant12 : Constant  Value=ENUM_SHIFTCOMMAND_D
  Constant13 : Constant  Value=ENUM_SHIFTCOMMAND_N
  Constant14 : Constant  Value=ENUM_PWRSTASW_READY
  Constant16 : Constant  Value=ENUM_CHRGPLUGSTA_NONE
  Constant17 : Constant  Value=ENUM_POWERSTA_STANDBY
  Constant18 : Constant  Value=ENUM_POWERSTA_ON
  Constant19 : Constant  Value=ENUM_POWERSTA_READY
  Constant2 : Constant  Value=ENUM_GEARSHIFTCMD_N
  Constant23 : Constant  Value=ENUM_PWRSTASW_STANDBY
  Constant24 : Constant  Value=ENUM_PWRSTASW_ON
  Constant25 : Constant  Value=ENUM_PWRSTASW_READY
  Constant26 : Constant  Value=KTQD_ForcePLimitSpd_kph
  Constant3 : Constant  Value=ENUM_GEARSHIFTCMD_P
  Constant4 : Constant  Value=ENUM_GEARSHIFTCMD_D
  Constant5 : Constant  Value=ENUM_SHIFTCOMMAND_P
  Constant6 : Constant  Value=ENUM_GEARSHIFTCMD_NONE
  Constant7 : Constant  Value=ENUM_GEARSHIFTCMD_P
  Constant8 : Constant  Value=ENUM_SHIFTCOMMAND_R
  Detect Change : simulink/Logic and Bit Operations/Detect Change  vinit=0  OutDataTypeStr=boolean
  Equal{,1..7,9,12..13,15} (12 alike) : RelationalOperator  Operator===  OutDataTypeStr=boolean  RndMeth=Simplest
  Equal14 : RelationalOperator  Operator=~=  OutDataTypeStr=boolean  RndMeth=Simplest
  Latch : hcu_lib/Basic_Blocks/Latch
  OR : Logic  Operator=OR  Inputs=3  AllPortsSameDT=off  OutDataTypeStr=boolean
  OR8 : Logic  Operator=OR  Inputs=3  AllPortsSameDT=off  OutDataTypeStr=boolean
  Relational Operator2 : RelationalOperator  Operator=<=  OutDataTypeStr=boolean  RndMeth=Simplest
  SR_Latch1 : hcu_lib/Basic_Blocks/SR_Latch
  Switch{,1..4} (5 alike) : Switch  Criteria=u2 ~= 0
      Switch1 settings: AttributesFormatString=%<Criteria>
      Switch2 settings: AttributesFormatString=%<Criteria>
      Switch3 settings: AttributesFormatString=%<Criteria>
      Switch4 settings: AttributesFormatString=%<Criteria>
  VTQD_GearShiftCMD_enum : Outport
  VTQD_PwrStaAllowPN_flg : Outport  Port=2
  VTQD_PwrStaAllowDR_flg : Outport  Port=3
  VTQD_ForceP_flg : Outport  Port=4
  wires:
  Switch2/1 -> Switch4/3
  Constant2/1 -> Switch4/1
  Switch1/1 -> Switch2/3
  [P] -> Switch2/2
  Constant3/1 -> Switch2/1
  Switch3/1 -> Switch1/3
  Constant/1 -> Switch3/1
  Constant4/1 -> Switch1/1
  [R] -> Switch3/2
  [D] -> Switch1/2
  VINP_ShifterHandleCmd_enum/1 -> [VINP_ShifterHandleCmd_enum]
  Constant5/1 -> Equal/2
  Constant8/1 -> Equal1/2
  Constant12/1 -> Equal2/2
  Constant19/1 -> Equal6/2
  [VPMM_PowerSta_enum] -> Equal6/1
  [VPMM_PowerSta_enum] -> Equal5/1
  [VPMM_PowerSta_enum] -> Equal4/1
  Constant17/1 -> Equal4/2
  Constant18/1 -> Equal5/2
  VPMM_PowerSta_enum/1 -> [VPMM_PowerSta_enum]
  Equal5/1 -> OR/2
  Equal4/1 -> OR/1
  Equal6/1 -> OR/3
  OR/1 -> VTQD_PwrStaAllowPN_flg/1  "VTQD_PwrStaAllowPN_flg"
  [VPMM_PowerSta_enum] -> Equal7/1
  Constant1/1 -> Equal7/2
  Equal7/1 -> VTQD_PwrStaAllowDR_flg/1  "VTQD_PwrStaAllowDR_flg"
  Equal/1 -> [P]
  Equal1/1 -> [R]
  Equal2/1 -> [D]
  Constant6/1 -> Switch3/3
  Switch/1 -> VTQD_GearShiftCMD_enum/1  "VTQD_GearShiftCMD_enum"
  Switch4/1 -> Switch/3
  [VTQD_ForceP_flg] -> Switch/2
  Constant7/1 -> Switch/1
  [VINP_ShifterHandleCmd_enum] -> Equal/1
  [VINP_ShifterHandleCmd_enum] -> Equal1/1
  [VINP_ShifterHandleCmd_enum] -> Equal2/1
  VINP_VehSpeed_kph/1 -> [VINP_VehSpeed_kph]
  VINP_ChrgPlugSta_enum/1 -> [VINP_ChrgPlugSta_enum]
  [VPMM_PowerSta_enum] -> Equal15/1
  [VINP_VehSpeed_kph] -> Relational Operator2/1
  Constant16/1 -> Equal14/2
  Equal12/1 -> OR8/2
  Equal15/1 -> OR8/1
  Constant23/1 -> Equal15/2
  Constant25/1 -> Equal13/2
  Constant26/1 -> Relational Operator2/2
  [VPMM_PowerSta_enum] -> Equal13/1
  Constant24/1 -> Equal12/2
  Equal13/1 -> OR8/3
  [VINP_ChrgPlugSta_enum] -> Equal14/1
  Equal14/1 -> AND5/1
  [VPMM_PowerSta_enum] -> Equal12/1
  AND5/1 -> SR_Latch1/1
  [VINP_ShifterHandleCmd_enum] -> Detect Change/1
  Constant13/1 -> Equal9/2
  [VINP_ShifterHandleCmd_enum] -> Equal9/1
  Equal9/1 -> [N]
  [N] -> Switch4/2
  Detect Change/1 -> SR_Latch1/2
  [VPMM_PowerSta_enum] -> Equal3/1
  Equal3/1 -> Latch/1
  Latch/1 -> AND5/2
  Constant14/1 -> Equal3/2
  Relational Operator2/1 -> AND5/3
  OR8/1 -> AND5/4
  SR_Latch1/1 -> [VTQD_ForceP_flg], VTQD_ForceP_flg/1  "VTQD_ForceP_flg"

== system tqd/TQD/TorqueDemand/ShiftModule/P_Button_State_Judge ==
  VINP_ShifterHandleCmd_enum : Inport
  Constant1 : Constant  Value=ENUM_PBUTTON_RELEASED
  Constant12 : Constant  Value=ENUM_SHIFTCOMMAND_D
  Constant15 : Constant  Value=ENUM_SHIFTCOMMAND_N
  Constant2 : Constant  Value=ENUM_PBUTTON_PRESSED
  Constant3 : Constant  Value=ENUM_PBUTTON_INVALID
  Constant4 : Constant  Value=ENUM_SHIFTCOMMAND_NONE
  Constant5 : Constant  Value=ENUM_SHIFTCOMMAND_P
  Constant8 : Constant  Value=ENUM_SHIFTCOMMAND_R
  Equal{,1..4} (5 alike) : RelationalOperator  Operator===  OutDataTypeStr=boolean  RndMeth=Simplest
  Logical Operator : Logic  Operator=OR  Inputs=4  AllPortsSameDT=off  OutDataTypeStr=boolean
  Switch1 : Switch  Criteria=u2 ~= 0
      settings: AttributesFormatString=%<Criteria>
  Switch4 : Switch  Criteria=u2 ~= 0
      settings: AttributesFormatString=%<Criteria>
  VTQD_PButtonSta_enum : Outport
  wires:
  Switch4/1 -> VTQD_PButtonSta_enum/1  "VTQD_PButtonSta_enum"
  VINP_ShifterHandleCmd_enum/1 -> [VINP_ShifterHandleCmd_enum]
  Equal/1 -> [P]
  Constant12/1 -> Equal2/2
  [VINP_ShifterHandleCmd_enum] -> Equal1/1
  Constant8/1 -> Equal1/2
  [VINP_ShifterHandleCmd_enum] -> Equal/1
  Equal2/1 -> Logical Operator/3
  Constant15/1 -> Equal3/2
  Equal3/1 -> Logical Operator/2
  Equal1/1 -> Logical Operator/1
  Constant5/1 -> Equal/2
  [VINP_ShifterHandleCmd_enum] -> Equal3/1
  [VINP_ShifterHandleCmd_enum] -> Equal2/1
  Logical Operator/1 -> [RND]
  [RND] -> Switch4/2
  [P] -> Switch1/2
  Constant1/1 -> Switch4/1
  Switch1/1 -> Switch4/3
  Constant2/1 -> Switch1/1
  Constant3/1 -> Switch1/3
  [VINP_ShifterHandleCmd_enum] -> Equal4/1
  Constant4/1 -> Equal4/2
  Equal4/1 -> Logical Operator/4

== system tqd/TQD/TorqueDemand/ShiftModule/SR_Latch1 ==
  set : Inport
  reset : Inport  Port=2
  Logical Operator : Logic  AllPortsSameDT=off  OutDataTypeStr=boolean
  Logical Operator1 : Logic  Operator=NOT  AllPortsSameDT=off  OutDataTypeStr=boolean
  Switch1 : Switch  Criteria=u2 ~= 0  Threshold=0.5
      settings: AttributesFormatString=<Criteria=%<Criteria>>
  Switch2 : Switch  Criteria=u2 ~= 0  Threshold=0.5
      settings: AttributesFormatString=<Criteria=%<Criteria>>
  Unit Delay : UnitDelay  SampleTime=-1  HasFrameUpgradeWarning=on
  latched : Outport
  wires:
  Switch1/1 -> Unit Delay/1, latched/1
  set/1 -> Switch1/1, Logical Operator/1
  reset/1 -> Switch2/2, Logical Operator1/1
  Unit Delay/1 -> Switch2/3
  Switch2/1 -> Switch1/3
  Logical Operator/1 -> Switch1/2
  Logical Operator1/1 -> Logical Operator/2, Switch2/1

== system tqd/TQD/TorqueDemand/Signal_convert/AWDMCUReadyExt_flg ==
  VINP_FrMCUErr_enum : Inport
  VINP_RrMCUErr_enum : Inport  Port=2
  Action Port : ActionPort
  Constant : Constant  Value=ENUM_MCUWARN_LV0
  Constant1 : Constant  Value=ENUM_MCUWARN_NOERROR
  Constant2 : Constant  Value=ENUM_MCUWARN_LV0
  Constant3 : Constant  Value=ENUM_MCUWARN_NOERROR
  Equal{,1..3} (4 alike) : RelationalOperator  Operator===  OutDataTypeStr=boolean  RndMeth=Simplest
  Logical Operator : Logic  Operator=OR  AllPortsSameDT=off  OutDataTypeStr=boolean
  Logical Operator1 : Logic  Operator=OR  AllPortsSameDT=off  OutDataTypeStr=boolean
  Logical Operator2 : Logic  AllPortsSameDT=off  OutDataTypeStr=boolean
  VTQD_AWDMCUReadyExt_flg : Outport
  wires:
  Logical Operator2/1 -> VTQD_AWDMCUReadyExt_flg/1
  Equal1/1 -> Logical Operator/2
  Equal/1 -> Logical Operator/1
  Constant1/1 -> Equal1/2
  VINP_FrMCUErr_enum/1 -> Equal1/1, Equal/1
  Constant/1 -> Equal/2
  Equal3/1 -> Logical Operator1/2
  Equal2/1 -> Logical Operator1/1
  Constant3/1 -> Equal3/2
  VINP_RrMCUErr_enum/1 -> Equal3/1, Equal2/1
  Constant2/1 -> Equal2/2
  Logical Operator/1 -> Logical Operator2/1
  Logical Operator1/1 -> Logical Operator2/2

== system tqd/TQD/TorqueDemand/Signal_convert/FWDMCUReadyExt_flg ==
  VINP_FrMCUErr_enum : Inport
  Action Port : ActionPort
  Constant : Constant  Value=ENUM_MCUWARN_LV0
  Constant1 : Constant  Value=ENUM_MCUWARN_NOERROR
  Equal : RelationalOperator  Operator===  OutDataTypeStr=boolean  RndMeth=Simplest
  Equal1 : RelationalOperator  Operator===  OutDataTypeStr=boolean  RndMeth=Simplest
  Logical Operator : Logic  Operator=OR  AllPortsSameDT=off  OutDataTypeStr=boolean
  VTQD_FWDMCUReadyExt_flg : Outport
  wires:
  Logical Operator/1 -> VTQD_FWDMCUReadyExt_flg/1
  Equal/1 -> Logical Operator/1
  VINP_FrMCUErr_enum/1 -> Equal1/1, Equal/1
  Constant/1 -> Equal/2
  Constant1/1 -> Equal1/2
  Equal1/1 -> Logical Operator/2

== system tqd/TQD/TorqueDemand/Signal_convert/RWDMCUReadyExt_flg ==
  VINP_RrMCUErr_enum : Inport
  Action Port : ActionPort
  Constant : Constant  Value=ENUM_MCUWARN_LV0
  Constant1 : Constant  Value=ENUM_MCUWARN_NOERROR
  Equal : RelationalOperator  Operator===  OutDataTypeStr=boolean  RndMeth=Simplest
  Equal1 : RelationalOperator  Operator===  OutDataTypeStr=boolean  RndMeth=Simplest
  Logical Operator : Logic  Operator=OR  AllPortsSameDT=off  OutDataTypeStr=boolean
  VTQD_RWDMCUReadyExt_flg : Outport
  wires:
  Logical Operator/1 -> VTQD_RWDMCUReadyExt_flg/1
  VINP_RrMCUErr_enum/1 -> Equal1/1, Equal/1
  Equal1/1 -> Logical Operator/2
  Equal/1 -> Logical Operator/1
  Constant1/1 -> Equal1/2
  Constant/1 -> Equal/2

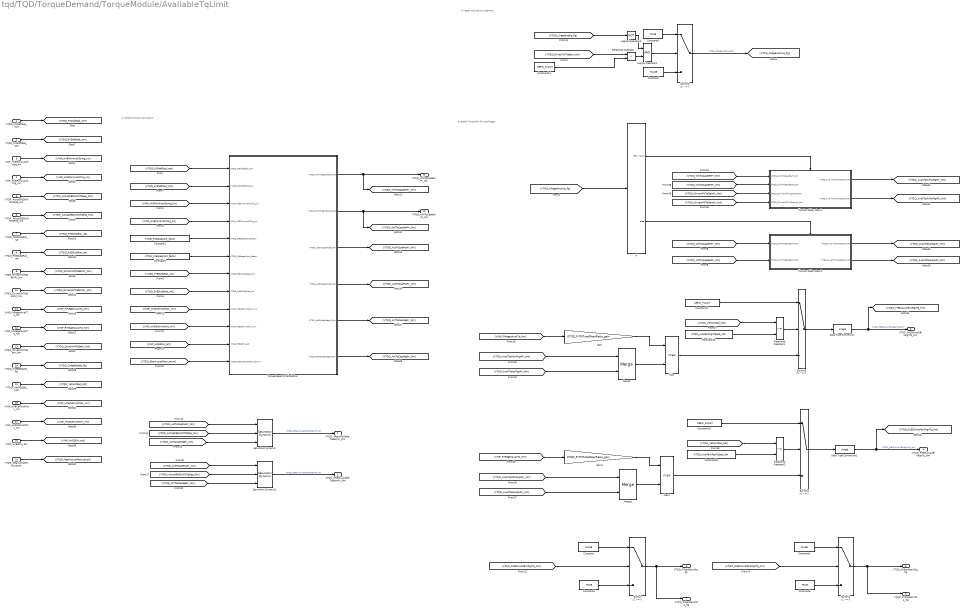
== system tqd/TQD/TorqueDemand/TorqueModule/AvaliableTqLimit ==
  note: Avaiable Torque for B-type Regen
  note: Available Torque Calculation
  note: A-regen activation judgment
  VTQD_FrShaftSpd_rpm : Inport
  VTQD_RrShaftSpd_rpm : Inport  Port=2
  VINP_HVBPwrAvailDchrg_kw : Inport  Port=3
  VINP_HVBPwrAvailChrg_kw : Inport  Port=4
  VTQR_ActualFEDUWhlTqReq_Nm : Inport  Port=5
  VTQR_ActualREDUWhlTqReq_Nm : Inport  Port=6
  VTQD_FrEDUSpRat_rat : Inport  Port=7
  VTQD_RrEDUSpRat_rat : Inport  Port=8
  VTQD_DriverWhlTqDemFr_Nm : Inport  Port=9
  VTQD_DriverWhlTqDemRr_Nm : Inport  Port=10
  VINP_FrRegenAvailTq_Nm : Inport  Port=11
  VINP_RrRegenAvailTq_Nm : Inport  Port=12
  VTQD_DriverWhlTqDem_Nm : Inport  Port=13
  VTQD_CreepEnable_flg : Inport  Port=14
  VTQD_VehActSpd_kph : Inport  Port=15
  VINP_HVBCellVoltMax_mV : Inport  Port=16
  VINP_HVBCellVoltMin_mV : Inport  Port=17
  VINP_HVBSOH_pct : Inport  Port=18
  VTQD_GearActualPosn_enum : Inport  Port=19
  Constant : Constant  Value=FALSE
  Constant14 : Constant  Value=ZERO_FLOAT
  Constant15 : Constant  Value=KTQD_AvailBrkRgnTqSpd_kph
  Constant17 : Constant  Value=ZERO_FLOAT
  Constant18 : Constant  Value=KTQD_AvailBrkRgnTqSpd_kph
  Constant2 : Constant  Value=KTQD_FrBatapCont_factor
  Constant20 : Constant  Value=ZERO_FLOAT
  Constant3 : Constant  Value=TRUE
  Constant4 : Constant  Value=FALSE
  Constant5 : Constant  Value=KTQD_RrBatapCont_factor
  Constant6 : Constant  Value=TRUE
  Constant7 : Constant  Value=FALSE
  Constant8 : Constant  Value=TRUE
  Data Type Conversion : DataTypeConversion  OutDataTypeStr=single
  Data Type Conversion1 : DataTypeConversion  OutDataTypeStr=single
  Gain : Gain  Gain=KTQD_FrTMTotalGearRatio_gain
  Gain1 : Gain  Gain=KTQD_RrTMTotalGearRatio_gain
  If : If  IfExpression=u1 ~= 0
  If Action Subsystem1 : Subsystem  TreatAsAtomicUnit=on
  If Action Subsystem2 : Subsystem  TreatAsAtomicUnit=on
  Logical Operator1 : Logic  AllPortsSameDT=off  OutDataTypeStr=boolean
  Logical Operator2 : Logic  Operator=NOT  AllPortsSameDT=off  OutDataTypeStr=boolean
  Max : MinMax  Function=max  Inputs=2
  Max1 : MinMax  Function=max  Inputs=2
  Merge : Merge
  Merge1 : Merge
  Relational Operator : RelationalOperator  Operator=<  OutDataTypeStr=boolean  RndMeth=Simplest
  Relational Operator1 : RelationalOperator  Operator=<=  OutDataTypeStr=boolean  RndMeth=Simplest
  Relational Operator2 : RelationalOperator  Operator=<=  OutDataTypeStr=boolean  RndMeth=Simplest
  Saturation Dynamic : simulink/Discontinuities/Saturation Dynamic  OutMin=[]  OutMax=[]  OutDataTypeStr=Inherit: Same as second input  OutDataType=fixdt(1, 16)  OutScaling=2^-10  DoSatur=off
  Saturation Dynamic1 : simulink/Discontinuities/Saturation Dynamic  OutMin=[]  OutMax=[]  OutDataTypeStr=Inherit: Same as second input  OutDataType=fixdt(1, 16)  OutScaling=2^-10  DoSatur=off
  Switch : Switch
  Switch1 : Switch
  Switch2 : Switch  Criteria=u2 ~= 0
  Switch3 : Switch  Criteria=u2 ~= 0
  Switch4 : Switch  Criteria=u2 ~= 0
  TorqueCapacityCalcalation : Subsystem
  VTQD_AfterAvailableTqDemFr_Nm : Outport
  VTQD_AfterAvailableTqDemRr_Nm : Outport  Port=2
  VTQD_FrEDUAvailBrkRgnTq_Nm : Outport  Port=3
  VTQD_RrEDUAvailBrkRgnTq_Nm : Outport  Port=4
  VTQD_FrRgnDecrSta_flg : Outport  Port=5
  VTQD_RrRgnDecrSta_flg : Outport  Port=6
  VTQD_FrRgnPermSta_flg : Outport  Port=7
  VTQD_RrRgnPermSta_flg : Outport  Port=8
  VTQD_WhlTqCapGenFr_Nm : Outport  Port=9
  VTQD_WhlTqCapGenRr_Nm : Outport  Port=10
  wires:
  VINP_FrRegenAvailTq_Nm/1 -> [VINP_FrRegenAvailTq_Nm]
  VINP_RrRegenAvailTq_Nm/1 -> [VINP_RrRegenAvailTq_Nm]
  Merge1/1 -> Max1/2
  [VINP_RrRegenAvailTq_Nm] -> Gain1/1
  Gain1/1 -> Max1/1
  Gain/1 -> Max/1
  Merge/1 -> Max/2
  [VINP_FrRegenAvailTq_Nm] -> Gain/1
  [VTQD_ARegenActive_flg] -> If/1
  Switch1/1 -> VTQD_RrRgnDecrSta_flg/1, VTQD_RrRgnPermSta_flg/1
  Constant6/1 -> Switch1/3
  Constant4/1 -> Switch1/1
  [VTQD_RrEDUAvailBrkRgnTq_Nm] -> Switch1/2
  Switch/1 -> VTQD_FrRgnDecrSta_flg/1, VTQD_FrRgnPermSta_flg/1
  Constant3/1 -> Switch/3
  Constant/1 -> Switch/1
  [VTQD_FrEDUAvailBrkRgnTq_Nm] -> Switch/2
  If/2 -> If Action Subsystem2/Action
  If/1 -> If Action Subsystem1/Action
  Data Type Conversion1/1 -> VTQD_RrEDUAvailBrkRgnTq_Nm/1, [VTQD_RrEDUAvailBrkRgnTq_Nm]  "VTQD_RrEDUAvailBrkRgnTq_Nm"
  Data Type Conversion/1 -> VTQD_FrEDUAvailBrkRgnTq_Nm/1, [VTQD_FrEDUAvailBrkRgnTq_Nm]  "VTQD_FrEDUAvailBrkRgnTq_Nm"
  VTQD_RrShaftSpd_rpm/1 -> [VTQD_RrShaftSpd_rpm]
  [VTQD_RrEDUSpRat_rat] -> TorqueCapacityCalcalation/8(VTQD_RrEDUSpRat_rat)
  [VTQD_FrEDUSpRat_rat] -> TorqueCapacityCalcalation/7(VTQD_FrEDUSpRat_cmd)
  Constant5/1 -> TorqueCapacityCalcalation/6(KTQD_RrBatapCont_factor)
  [VTQD_RrShaftSpd_rpm] -> TorqueCapacityCalcalation/2(VTQD_RrShaftSpd_rpm)
  Constant2/1 -> TorqueCapacityCalcalation/5(KTQD_FrBatapCont_factor)
  [VINP_HVBPwrAvailChrg_kw] -> TorqueCapacityCalcalation/4(VINP_HVBPwrAvailChrg_kw)
  [VINP_HVBPwrAvailDchrg_kw] -> TorqueCapacityCalcalation/3(VINP_HVBPwrAvailDchrg_kw)
  [VTQD_FrShaftSpd_rpm] -> TorqueCapacityCalcalation/1(VTQD_FrShaftSpd_rpm)
  TorqueCapacityCalcalation/1(VTQD_WhlTqCapGenFr_Nm) -> [VTQD_WhlTqCapGenFr_Nm], VTQD_WhlTqCapGenFr_Nm/1
  If Action Subsystem2/2(VTQD_AvailTqNoARgnRr_Nm) -> [VTQD_AvailTqNoARgnRr_Nm]
  If Action Subsystem2/1(VTQD_AvailTqNoARgnFr_Nm) -> [VTQD_AvailTqNoARgnFr_Nm]
  [VTQD_WhlTqCapGenRr_Nm] -> If Action Subsystem2/2(VTQD_WhlTqCapGenR_Nm)
  [VTQD_WhlTqCapGenFr_Nm] -> If Action Subsystem2/1(VTQD_WhlTqCapGenF_Nm)
  [VTQD_WhlTqCapGenRr_Nm] -> If Action Subsystem1/2(VTQD_WhlTqCapGenR_Nm)
  [VTQD_WhlTqCapGenFr_Nm] -> If Action Subsystem1/1(VTQD_WhlTqCapGenF_Nm)
  [VTQD_DriverWhlTqDemRr_Nm] -> If Action Subsystem1/4(VTQD_DriverWhlTqDemRr_Nm)
  [VTQD_DriverWhlTqDemFr_Nm] -> If Action Subsystem1/3(VTQD_DriverWhlTqDemFr_Nm)
  VTQD_DriverWhlTqDemRr_Nm/1 -> [VTQD_DriverWhlTqDemRr_Nm]
  VTQD_DriverWhlTqDemFr_Nm/1 -> [VTQD_DriverWhlTqDemFr_Nm]
  VTQD_RrEDUSpRat_rat/1 -> [VTQD_RrEDUSpRat_rat]
  VTQD_FrEDUSpRat_rat/1 -> [VTQD_FrEDUSpRat_rat]
  VTQR_ActualREDUWhlTqReq_Nm/1 -> [VTQR_ActualREDUWhlTqReq_Nm]
  VTQR_ActualFEDUWhlTqReq_Nm/1 -> [VTQR_ActualFEDUWhlTqReq_Nm]
  VINP_HVBPwrAvailDchrg_kw/1 -> [VINP_HVBPwrAvailDchrg_kw]
  VTQD_FrShaftSpd_rpm/1 -> [VTQD_FrShaftSpd_rpm]
  VINP_HVBPwrAvailChrg_kw/1 -> [VINP_HVBPwrAvailChrg_kw]
  Switch2/1 -> [VTQD_ARegenActive_flg]  "VTQD_ARegenActive_flg"
  VTQD_DriverWhlTqDem_Nm/1 -> [VTQD_DriverWhlTqDem_Nm]
  VTQD_CreepEnable_flg/1 -> [VTQD_CreepEnable_flg]
  [VTQD_CreepEnable_flg] -> Logical Operator2/1
  Logical Operator1/1 -> Switch2/2
  [VTQD_DriverWhlTqDem_Nm] -> Relational Operator/1
  Relational Operator/1 -> Logical Operator1/2
  Constant14/1 -> Relational Operator/2
  Constant7/1 -> Switch2/3
  Constant8/1 -> Switch2/1
  Logical Operator2/1 -> Logical Operator1/1
  Constant17/1 -> Switch3/1
  Relational Operator1/1 -> Switch3/2
  Constant15/1 -> Relational Operator1/2
  Max/1 -> Switch3/3
  Switch3/1 -> Data Type Conversion/1
  Constant20/1 -> Switch4/1
  Max1/1 -> Switch4/3
  Relational Operator2/1 -> Switch4/2
  Constant18/1 -> Relational Operator2/2
  Switch4/1 -> Data Type Conversion1/1
  [VTQD_AvailTqNoARgnRr_Nm] -> Merge1/2
  [VTQD_AvailTqWithARgnRr_Nm] -> Merge1/1
  [VTQD_AvailTqNoARgnFr_Nm] -> Merge/2
  [VTQD_AvailTqWithARgnFr_Nm] -> Merge/1
  Saturation Dynamic/1 -> VTQD_AfterAvailableTqDemFr_Nm/1  "VTQD_AfterAvailableTqDemFr_Nm"
  Saturation Dynamic1/1 -> VTQD_AfterAvailableTqDemRr_Nm/1  "VTQD_AfterAvailableTqDemRr_Nm"
  [VTQD_ActTqCapPosFr_Nm] -> Saturation Dynamic/1
  [VTQD_ActTqCapPosRr_Nm] -> Saturation Dynamic1/1
  VTQD_VehActSpd_kph/1 -> [VTQD_VehActSpd_kph]
  [VTQD_VehActSpd_kph] -> Relational Operator1/1
  [VTQD_VehActSpd_kph] -> Relational Operator2/1
  [VTQD_ActTqCapNegFr_Nm] -> Saturation Dynamic/3
  [VTQD_ActTqCapNegRr_Nm] -> Saturation Dynamic1/3
  VINP_HVBCellVoltMin_mV/1 -> [VINP_HVBCellVoltMin_mV]
  VINP_HVBSOH_pct/1 -> [VINP_HVBSOH_pct]
  VINP_HVBCellVoltMax_mV/1 -> [VINP_HVBCellVoltMax_mV]
  [VINP_HVBCellVoltMax_mV] -> TorqueCapacityCalcalation/9(VINP_HVBCellVoltMax_mV)
  [VINP_HVBCellVoltMin_mV] -> TorqueCapacityCalcalation/10(VINP_HVBCellVoltMin_mV)
  [VINP_HVBSOH_pct] -> TorqueCapacityCalcalation/11(VINP_HVBSOH_pct)
  If Action Subsystem1/1(VTQD_AvailTqWithARgnFr_Nm) -> [VTQD_AvailTqWithARgnFr_Nm]
  If Action Subsystem1/2(VTQD_AvailTqWithARgnRr_Nm) -> [VTQD_AvailTqWithARgnRr_Nm]
  [VTQR_ActualFEDUWhlTqReq_Nm] -> Saturation Dynamic/2
  [VTQR_ActualREDUWhlTqReq_Nm] -> Saturation Dynamic1/2
  VTQD_GearActualPosn_enum/1 -> [VTQD_GearActualPosn_enum]
  [VTQD_GearActualPosn_enum] -> TorqueCapacityCalcalation/12(VTQD_GearActualPosn_enum)
  TorqueCapacityCalcalation/3(VTQD_ActTqCapPosFr_Nm) -> [VTQD_ActTqCapPosFr_Nm]
  TorqueCapacityCalcalation/4(VTQD_ActTqCapPosRr_Nm) -> [VTQD_ActTqCapPosRr_Nm]
  TorqueCapacityCalcalation/5(VTQD_ActTqCapNegFr_Nm) -> [VTQD_ActTqCapNegFr_Nm]
  TorqueCapacityCalcalation/6(VTQD_ActTqCapNegRr_Nm) -> [VTQD_ActTqCapNegRr_Nm]
  TorqueCapacityCalcalation/2(VTQD_WhlTqCapGenRr_Nm) -> [VTQD_WhlTqCapGenRr_Nm], VTQD_WhlTqCapGenRr_Nm/1
